simulink subsystem "LRLM_ECU"  (R2021a)
settings: Solver=VariableStepAuto  StartTime=0.0  StopTime=10.0  RelTol=1e-3
model mask{time_period=1}
  mask prompts: time_period "Enter the time period for the blinking lights (s)"
libraries: simulink x4
settings Model: Creator=Sai229  LastModifiedBy=Sai229

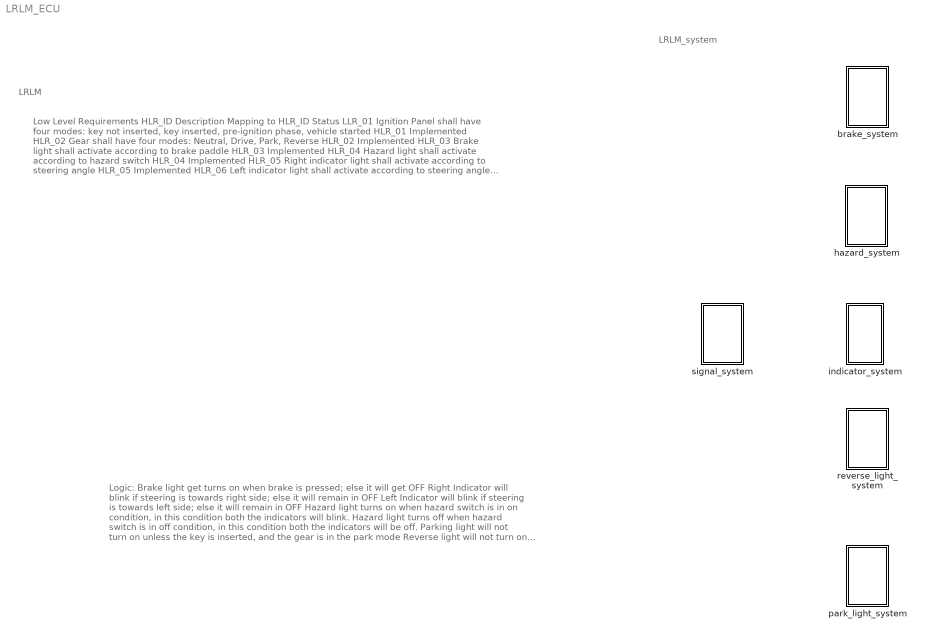
== system LRLM_ECU ==
  note: LRLM
  note: LRLM_system
  note: Low Level Requirements
      |
      | HLR_ID
      | Description
      | Mapping to HLR_ID
      | Status
      |
      | LLR_01
      | Ignition Panel shall have four modes: key not inserted, key inserted, pre-ignition phase, vehicle started
      | HLR_01
      | Implemented
      |
      | HLR_02
      | Gear shall have four modes: Neutral, Drive, Park, Reverse
      | HLR_02
      | Implemented
      |
      | HLR_03
      | Brake light shall activate according to brake paddle
      | HLR_03
      | Implemented
      |
      | HLR_04
      | Hazard light shall activate according to hazard switch
      | HLR_04
      | Implemented
      |
      | HLR_05
      | Right indicator light shall activate according to steering angle
      | HLR_05
      | Implemented
      |
      | HLR_06
      | Left indicator light shall activate according to steering angle
      | HLR_05
      | Implemented
      |
      | HLR_07
      | Parking light shall activate according to park gear
      | HLR_06
      | Implemented
      |
      | HLR_08
      | Reversing lights shall activate according to reverse gear
      | HLR_07
      | Implemented
  note: Logic:
      | Brake light get turns on when brake is pressed; else it will get OFF
      | Right Indicator will blink if steering is towards right side; else it will remain in OFF
      | Left Indicator will blink if steering is towards left side; else it will remain in OFF
      | Hazard light turns on when hazard switch is in on condition, in this condition both the indicators will blink.
      | Hazard light turns off when hazard switch is in off condition, in this condition both the indicators will be off.
      | Parking light will not turn on unless the key is inserted, and the gear is in the park mode
      | Reverse light will not turn on unless the key is inserted, and the gear is in the reverse mode
  brake_system : Subsystem
  hazard_system : Subsystem
  indicator_system : Subsystem
  park_light_system : Subsystem
  reverse_light_system : Subsystem
  signal_system : Subsystem

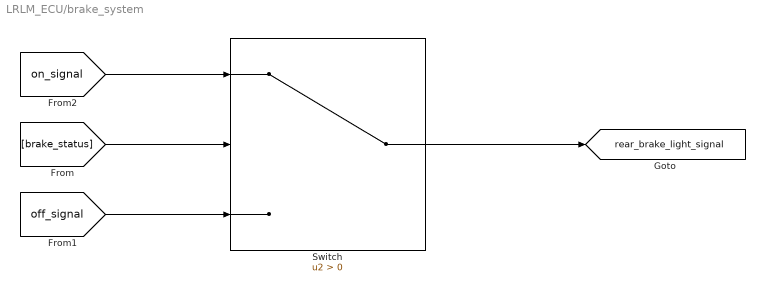
== system LRLM_ECU/brake_system ==
  Switch : Switch  Criteria=u2 > Threshold
  tag scope: rear_brake_light_signal=global
  wires:
  [brake_status] -> Switch/2
  [off_signal] -> Switch/3
  Switch/1 -> [rear_brake_light_signal]
  [on_signal] -> Switch/1

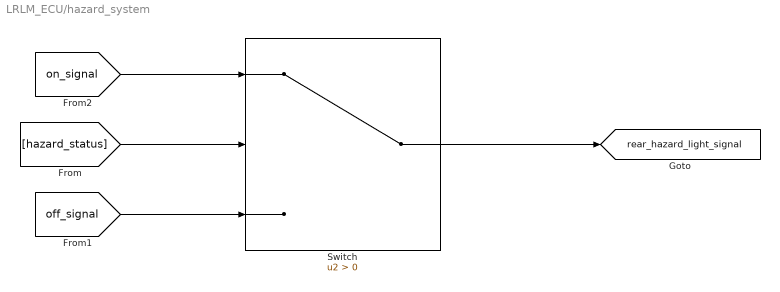
== system LRLM_ECU/hazard_system ==
  Switch : Switch  Criteria=u2 > Threshold
  tag scope: rear_hazard_light_signal=global
  wires:
  [on_signal] -> Switch/1
  Switch/1 -> [rear_hazard_light_signal]
  [off_signal] -> Switch/3
  [hazard_status] -> Switch/2

== system LRLM_ECU/indicator_system ==
  left_indicator_system : Subsystem
  right_indicator_system : Subsystem

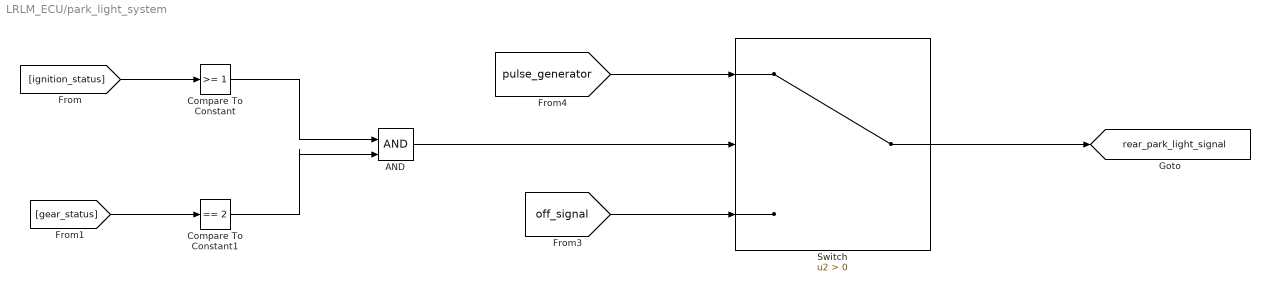
== system LRLM_ECU/park_light_system ==
  AND : Logic  IconShape=distinctive  AllPortsSameDT=off  OutDataTypeStr=boolean
  Compare To Constant : simulink/Logic and Bit Operations/Compare To Constant  relop=>=  const=1  OutDataTypeStr=boolean
  Compare To Constant1 : simulink/Logic and Bit Operations/Compare To Constant  relop===  const=2  OutDataTypeStr=boolean
  Switch : Switch  Criteria=u2 > Threshold
  tag scope: rear_park_light_signal=global
  wires:
  [off_signal] -> Switch/3
  Switch/1 -> [rear_park_light_signal]
  AND/1 -> Switch/2
  [pulse_generator] -> Switch/1
  [gear_status] -> Compare To Constant1/1
  [ignition_status] -> Compare To Constant/1
  Compare To Constant1/1 -> AND/2
  Compare To Constant/1 -> AND/1

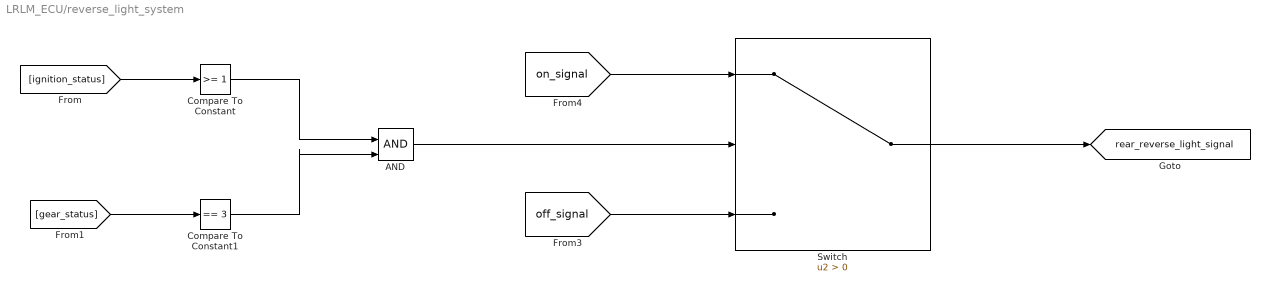
== system LRLM_ECU/reverse_light_system ==
  AND : Logic  IconShape=distinctive  AllPortsSameDT=off  OutDataTypeStr=boolean
  Compare To Constant : simulink/Logic and Bit Operations/Compare To Constant  relop=>=  const=1  OutDataTypeStr=boolean
  Compare To Constant1 : simulink/Logic and Bit Operations/Compare To Constant  relop===  const=3  OutDataTypeStr=boolean
  Switch : Switch  Criteria=u2 > Threshold
  tag scope: rear_reverse_light_signal=global
  wires:
  Compare To Constant/1 -> AND/1
  Compare To Constant1/1 -> AND/2
  [ignition_status] -> Compare To Constant/1
  [gear_status] -> Compare To Constant1/1
  [on_signal] -> Switch/1
  AND/1 -> Switch/2
  Switch/1 -> [rear_reverse_light_signal]
  [off_signal] -> Switch/3

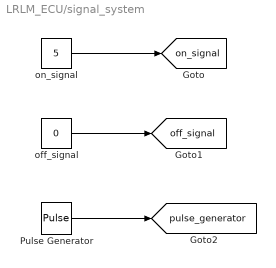
== system LRLM_ECU/signal_system ==
  Pulse Generator : DiscretePulseGenerator  PulseType=Time based  Amplitude=5  Period=time_period  PulseWidth=50
  off_signal : Constant  Value=0
  on_signal : Constant  Value=5
  tag scope: off_signal=global, on_signal=global, pulse_generator=global
  wires:
  Pulse Generator/1 -> [pulse_generator]
  off_signal/1 -> [off_signal]
  on_signal/1 -> [on_signal]

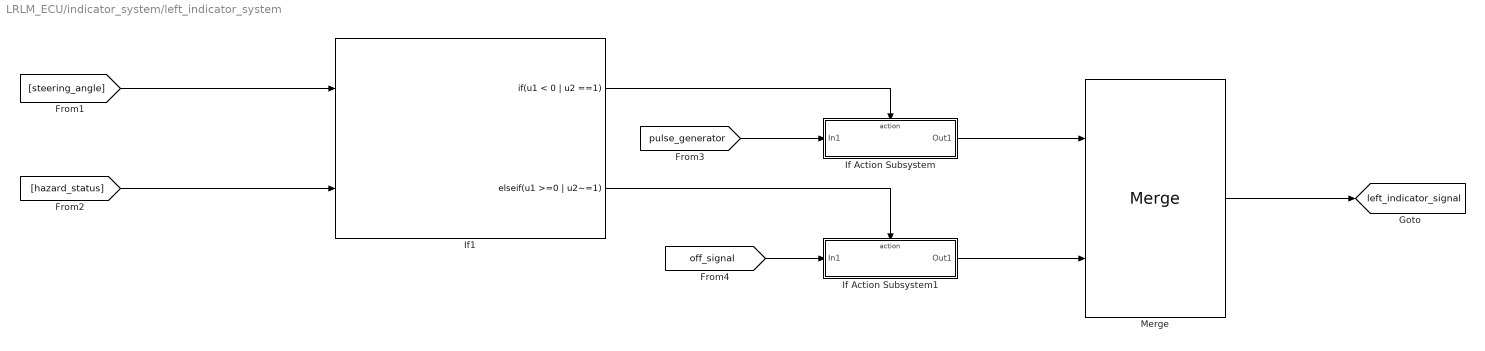
== system LRLM_ECU/indicator_system/left_indicator_system ==
  If Action Subsystem : Subsystem  TreatAsAtomicUnit=on
  If Action Subsystem1 : Subsystem  TreatAsAtomicUnit=on
  If1 : If  NumInputs=2  IfExpression=u1 < 0 | u2 ==1  ElseIfExpressions=u1 >=0 | u2~=1  ShowElse=off
  Merge : Merge
  tag scope: left_indicator_signal=global
  wires:
  [pulse_generator] -> If Action Subsystem/1(In1)
  [off_signal] -> If Action Subsystem1/1(In1)
  If1/1 -> If Action Subsystem/Action
  If Action Subsystem/1(Out1) -> Merge/1
  [steering_angle] -> If1/1
  [hazard_status] -> If1/2
  If Action Subsystem1/1(Out1) -> Merge/2
  If1/2 -> If Action Subsystem1/Action
  Merge/1 -> [left_indicator_signal]

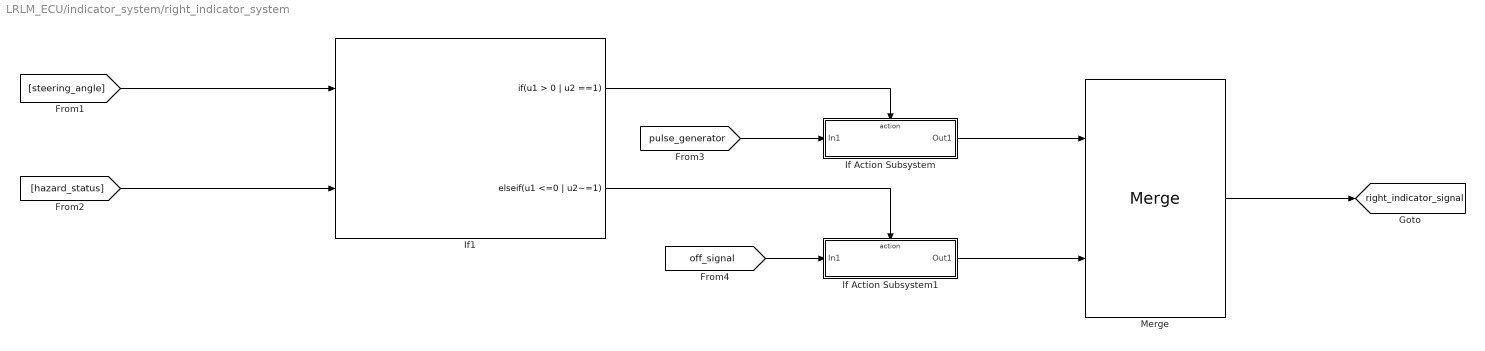
== system LRLM_ECU/indicator_system/right_indicator_system ==
  If Action Subsystem : Subsystem  TreatAsAtomicUnit=on
  If Action Subsystem1 : Subsystem  TreatAsAtomicUnit=on
  If1 : If  NumInputs=2  IfExpression=u1 > 0 | u2 ==1  ElseIfExpressions=u1 <=0 | u2~=1  ShowElse=off
  Merge : Merge
  tag scope: right_indicator_signal=global
  wires:
  Merge/1 -> [right_indicator_signal]
  [hazard_status] -> If1/2
  If Action Subsystem/1(Out1) -> Merge/1
  If1/2 -> If Action Subsystem1/Action
  If1/1 -> If Action Subsystem/Action
  [pulse_generator] -> If Action Subsystem/1(In1)
  [steering_angle] -> If1/1
  If Action Subsystem1/1(Out1) -> Merge/2
  [off_signal] -> If Action Subsystem1/1(In1)

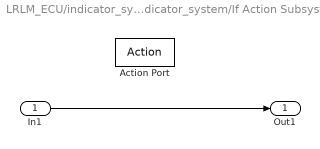
== system LRLM_ECU/indicator_system/left_indicator_system/If Action Subsystem ==
  In1 : Inport
  Action Port : ActionPort
  Out1 : Outport
  wires:
  In1/1 -> Out1/1

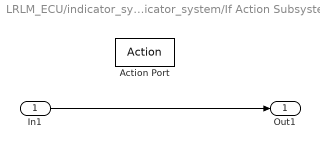
== system LRLM_ECU/indicator_system/left_indicator_system/If Action Subsystem1 ==
  In1 : Inport
  Action Port : ActionPort
  Out1 : Outport
  wires:
  In1/1 -> Out1/1

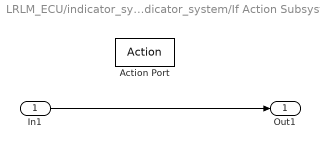
== system LRLM_ECU/indicator_system/right_indicator_system/If Action Subsystem ==
  In1 : Inport
  Action Port : ActionPort
  Out1 : Outport
  wires:
  In1/1 -> Out1/1

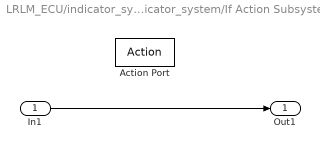
== system LRLM_ECU/indicator_system/right_indicator_system/If Action Subsystem1 ==
  In1 : Inport
  Action Port : ActionPort
  Out1 : Outport
  wires:
  In1/1 -> Out1/1
